simulink model "doc_convinterleaver"  (R2014a)
settings: Solver=ode45  StartTime=0.0  StopTime=20  RelTol=1e-3
undefined symbols (not defined in the file or in its folder): commblksprivate, Info
libraries: commcnvintrlv2 x2, simulink x1
settings Model: Creator=The MathWorks Inc.
settings DataIOCC: SignalLoggingSaveFormat=ModelDataLogs
settings OptimizationCC: BlockReduction=off  BooleanDataType=off  ExpressionDepthLimit=2147483647
settings DebuggingCC: SaveWithParameterizedLinksMsg=none  UnderspecifiedInitializationDetection=Classic  SignalResolutionControl=TryResolveAllWithWarning  SolverPrmCheckMsg=none  MultiTaskDSMMsg=warning  MultiTaskCondExecSysMsg=none  FcnCallInpInsideContextMsg=UseLocalSettings  StateNameClashWarn=warning  StrictBusMsg=None
settings HardwareCC: TargetUnknown=on
settings RTWCC: IncludeERTFirstTime=on
settings GRTTargetCC: CombineOutputUpdateFcns=off  GRTInterface=on

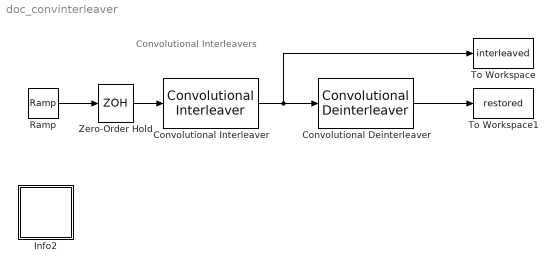
== system doc_convinterleaver ==
  note: Convolutional Interleavers
  Convolutional Deinterleaver : commcnvintrlv2/Convolutional Deinterleaver  N=3  B=2  ic=[-1 -2 -3]'
  Convolutional Interleaver : commcnvintrlv2/Convolutional Interleaver  N=3  B=2  ic=[-1 -2 -3]'
  Info2 : Subsystem  AncestorBlock=commblksprivate/Info  mask(Info){}
      settings: OpenFcn=helpview([docroot '/toolbox/comm/comm.map'], 'doc_convinterleaver')
      mask Display: disp('Info')
  Ramp : simulink/Sources/Ramp  slope=1  start=0  X0=0
  To Workspace : ToWorkspace  VariableName=interleaved  SampleTime=-1
  To Workspace1 : ToWorkspace  VariableName=restored  SampleTime=-1
  Zero-Order Hold : ZeroOrderHold
  wires:
  Ramp/1 -> Zero-Order Hold/1
  Zero-Order Hold/1 -> Convolutional Interleaver/1
  Convolutional Interleaver/1 -> Convolutional Deinterleaver/1, To Workspace/1
  Convolutional Deinterleaver/1 -> To Workspace1/1

== system doc_convinterleaver/Info2 ==
